simulink model "PAM"  (R2020a)
settings: Solver=VariableStepAuto  StartTime=0.0  StopTime=10.0  RelTol=1e-3
libraries: simulink_extras x1
settings Model: Creator=Admin  LastModifiedBy=fazal
settings SFSimCC: CustomCodeUndefinedFunction=UseInterfaceOnly

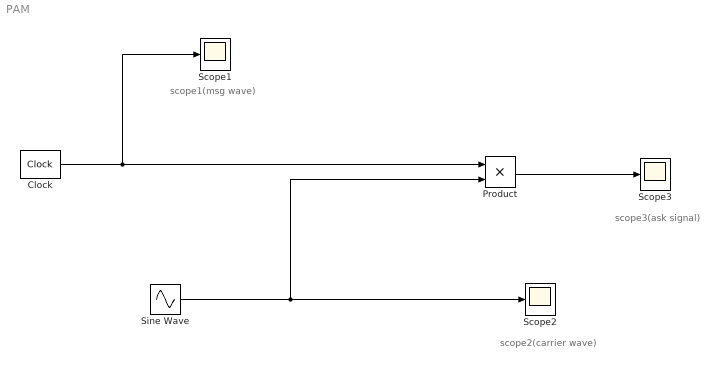
== system PAM ==
  note: scope1(msg wave)
  note: scope2(carrier wave)
  note: scope3(ask signal)
  Clock : simulink_extras/Flip Flops/Clock  period=0.2
  Product : Product
  Scope1 : Scope
  Scope2 : Scope
  Scope3 : Scope
  Sine Wave : Sin  Frequency=2  SampleTime=0.00002
  wires:
  Product/1 -> Scope3/1
  Sine Wave/1 -> Product/2, Scope2/1
  Clock/1 -> Scope1/1, Product/1
